simulink model "Q5"  (R2020b)
settings: Solver=VariableStepAuto  StartTime=0.0  StopTime=10.0  RelTol=1e-3
undefined symbols (not defined in the file): C, R
settings Model: Creator=HP  LastModifiedBy=HP

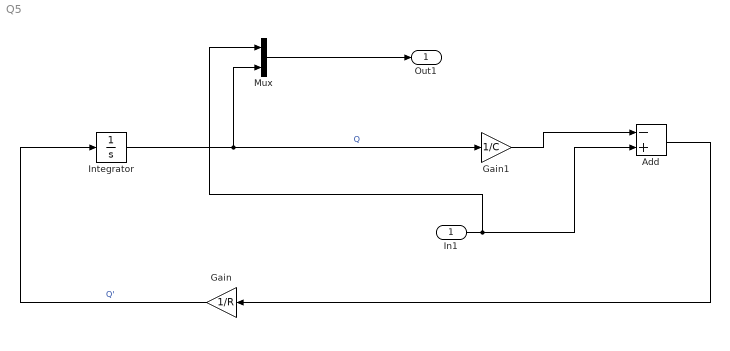
== system Q5 ==
  In1 : Inport
  Add : Sum  Inputs=-+
  Gain : Gain  Gain=1/R
  Gain1 : Gain  Gain=1/C
  Integrator : Integrator
  Mux : Mux  Inputs=2
  Out1 : Outport
  wires:
  Integrator/1 -> Gain1/1, Mux/2  "Q"
  Gain1/1 -> Add/1
  Gain/1 -> Integrator/1  "Q'"
  Add/1 -> Gain/1
  In1/1 -> Mux/1, Add/2
  Mux/1 -> Out1/1
